simulink model "DIAGRAMA MATLAB"  (R2016a)
settings: Solver=VariableStepAuto  StartTime=0.0  StopTime=20  RelTol=1e-3
settings Model: Creator=Willian  LastModifiedBy=Willian

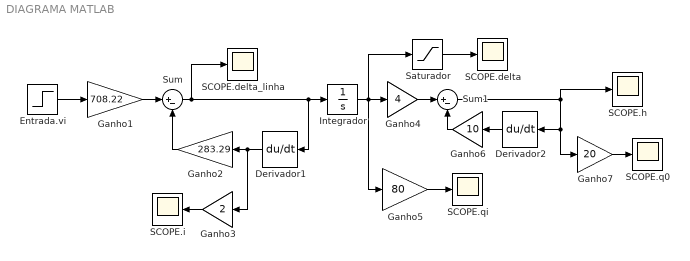
== system DIAGRAMA MATLAB ==
  Derivador1 : Derivative
  Derivador2 : Derivative
  Entrada.vi : Step  After=0.2  SampleTime=0
  Ganho1 : Gain  Gain=708.22
  Ganho2 : Gain  Gain=283.29
  Ganho3 : Gain  Gain=2
  Ganho4 : Gain  Gain=4
  Ganho5 : Gain  Gain=80
  Ganho6 : Gain  Gain=10
  Ganho7 : Gain  Gain=20
  Integrador : Integrator
  SCOPE.delta : Scope
  SCOPE.delta_linha : Scope
  SCOPE.h : Scope
  SCOPE.i : Scope
  SCOPE.q0 : Scope
  SCOPE.qi : Scope
  Saturador : Saturate  UpperLimit=2*pi  LowerLimit=0
  Sum : Sum  Inputs=|+-
  Sum1 : Sum  Inputs=|+-
  wires:
  Entrada.vi/1 -> Ganho1/1
  Ganho1/1 -> Sum/1
  Sum/1 -> Derivador1/1, Integrador/1, SCOPE.delta_linha/1
  Derivador1/1 -> Ganho3/1, Ganho2/1
  Ganho2/1 -> Sum/2
  Ganho3/1 -> SCOPE.i/1
  Integrador/1 -> Saturador/1, Ganho5/1, Ganho4/1
  Ganho5/1 -> SCOPE.qi/1
  Ganho4/1 -> Sum1/1
  Ganho7/1 -> SCOPE.q0/1
  Derivador2/1 -> Ganho6/1
  Ganho6/1 -> Sum1/2
  Saturador/1 -> SCOPE.delta/1
  Sum1/1 -> SCOPE.h/1, Derivador2/1, Ganho7/1
